simulink model "ex_harmonic_cancellation"  (R2022b)
settings: Solver=FixedStepDiscrete  StartTime=0.0  StopTime=0.3  FixedStep=0.001  RelTol=1e-3
settings Model: Creator=realj  LastModifiedBy=realj

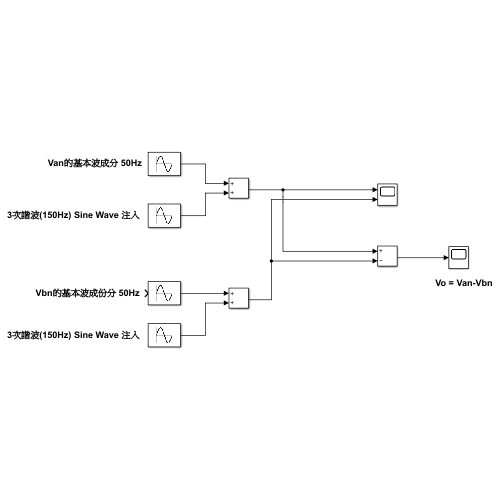
[thumbnail: Simulink's stored preview of the top-level diagram]
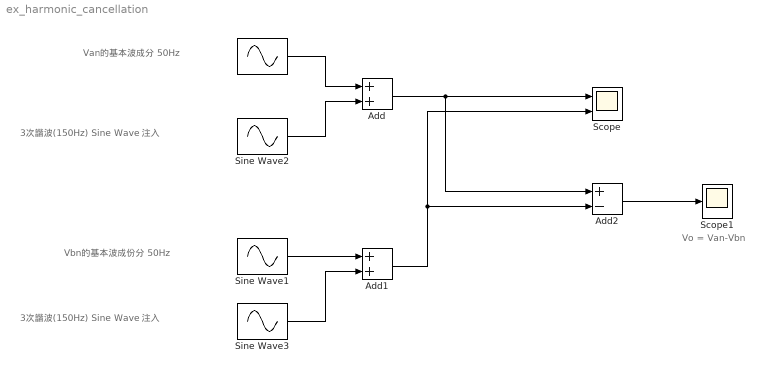
== system ex_harmonic_cancellation ==
  note: Van的基本波成分 50Hz
  note: 3次諧波(150Hz) Sine Wave 注入
  note: Vbn的基本波成份分 50Hz
  note: 3次諧波(150Hz) Sine Wave 注入
  note: Vo = Van-Vbn
  " " : Sin  Frequency=50  SampleTime=0
  Add : Sum
  Add1 : Sum
  Add2 : Sum  Inputs=+-
  Scope : Scope  NumInputPorts=2
  Scope1 : Scope
  Sine Wave1 : Sin  TimeSource=Use external signal  Frequency=50  Phase=pi  SampleTime=0
  Sine Wave2 : Sin  Frequency=150  SampleTime=0
  Sine Wave3 : Sin  Frequency=150  SampleTime=0
  wires:
  " "/1 -> Add/1
  Sine Wave2/1 -> Add/2
  Add/1 -> Add2/1, Scope/1
  Sine Wave1/1 -> Add1/1
  Sine Wave3/1 -> Add1/2
  Add1/1 -> Add2/2, Scope/2
  Add2/1 -> Scope1/1
